simulink model "HA1_model"  (R2015a)
settings: Solver=ode45  StartTime=0.0  StopTime=10.0  RelTol=1e-3
settings Model: Creator=adokhanc  LastModifiedBy=adokhanc
settings DebuggingCC: UnderspecifiedInitializationDetection=Classic  MergeDetectMultiDrivingBlocksExec=none  SolverPrmCheckMsg=warning  StateNameClashWarn=warning

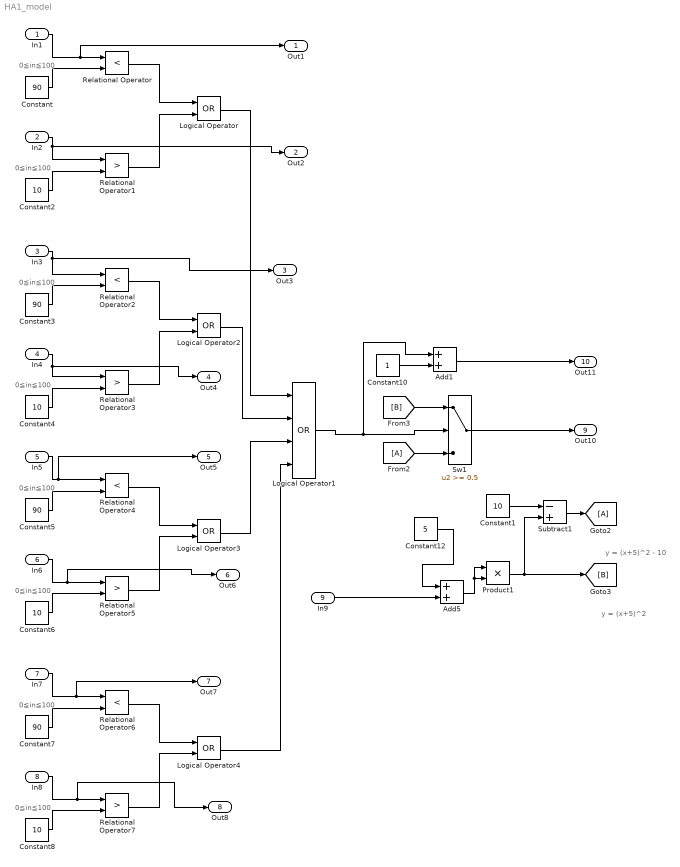
== system HA1_model ==
  note: 0≦in≦100
  note: 0≦in≦100
  note: 0≦in≦100
  note: 0≦in≦100
  note: 0≦in≦100
  note: 0≦in≦100
  note: 0≦in≦100
  note: 0≦in≦100
  note: y = (x+5)^2
  note: y = (x+5)^2 - 10
  In1 : Inport
  In2 : Inport  Port=2
  In3 : Inport  Port=3
  In4 : Inport  Port=4
  In5 : Inport  Port=5
  In6 : Inport  Port=6
  In7 : Inport  Port=7
  In8 : Inport  Port=8
  In9 : Inport  Port=9
  Add1 : Sum
  Add5 : Sum
  Constant{,3,5,7} (4 alike) : Constant  Value=90
  Constant{1..2,4,6,8} (5 alike) : Constant  Value=10
  Constant10 : Constant
  Constant12 : Constant  Value=5
  Logical Operator{,2..4} (4 alike) : Logic  Operator=OR  AllPortsSameDT=off  OutDataTypeStr=boolean
  Logical Operator1 : Logic  Operator=OR  Inputs=4  AllPortsSameDT=off  OutDataTypeStr=boolean
  Product1 : Product  RndMeth=Zero
  Relational Operator{,2,4,6} (4 alike) : RelationalOperator  Operator=<  OutDataTypeStr=boolean
  Relational Operator{1,3,5,7} (4 alike) : RelationalOperator  Operator=>  OutDataTypeStr=boolean
  Subtract1 : Sum  Inputs=-+
  Sw1 : Switch  Threshold=0.5  RndMeth=Simplest  InputSameDT=on
  "Out1 " : Outport
  Out2 : Outport  Port=2
  "Out3 " : Outport  Port=3
  Out4 : Outport  Port=4
  Out5 : Outport  Port=5
  Out6 : Outport  Port=6
  Out7 : Outport  Port=7
  Out8 : Outport  Port=8
  Out10 : Outport  Port=9
  Out11 : Outport  Port=10
  wires:
  [B] -> Sw1/1
  [A] -> Sw1/3
  Product1/1 -> Subtract1/2, [B]
  Constant1/1 -> Subtract1/1
  Subtract1/1 -> [A]
  Constant/1 -> Relational Operator/2
  Constant2/1 -> Relational Operator1/2
  Relational Operator/1 -> Logical Operator/1
  Relational Operator1/1 -> Logical Operator/2
  Constant3/1 -> Relational Operator2/2
  Constant4/1 -> Relational Operator3/2
  Relational Operator2/1 -> Logical Operator2/1
  Relational Operator3/1 -> Logical Operator2/2
  Constant5/1 -> Relational Operator4/2
  Constant6/1 -> Relational Operator5/2
  Relational Operator4/1 -> Logical Operator3/1
  Relational Operator5/1 -> Logical Operator3/2
  Constant7/1 -> Relational Operator6/2
  Constant8/1 -> Relational Operator7/2
  Relational Operator6/1 -> Logical Operator4/1
  Relational Operator7/1 -> Logical Operator4/2
  Logical Operator/1 -> Logical Operator1/1
  Logical Operator2/1 -> Logical Operator1/2
  Logical Operator3/1 -> Logical Operator1/3
  Logical Operator4/1 -> Logical Operator1/4
  In1/1 -> "Out1 "/1, Relational Operator/1
  In2/1 -> Relational Operator1/1, Out2/1
  In3/1 -> "Out3 "/1, Relational Operator2/1
  In4/1 -> Out4/1, Relational Operator3/1
  In5/1 -> Out5/1, Relational Operator4/1
  In6/1 -> Out6/1, Relational Operator5/1
  In7/1 -> Out7/1, Relational Operator6/1
  In8/1 -> Out8/1, Relational Operator7/1
  Constant10/1 -> Add1/2
  Sw1/1 -> Out10/1
  Add1/1 -> Out11/1
  Constant12/1 -> Add5/1
  Add5/1 -> Product1/2, Product1/1
  In9/1 -> Add5/2
  Logical Operator1/1 -> Add1/1, Sw1/2
